simulink model "sistemas_mecanicos_simulink_simscape"  (R2025b)
settings: Solver=ode23t  StartTime=0.0  StopTime=10  RelTol=1e-3
libraries: fl_lib x21, nesl_utility x8
settings Model: Creator=Lenovo  LastModifiedBy=Lenovo

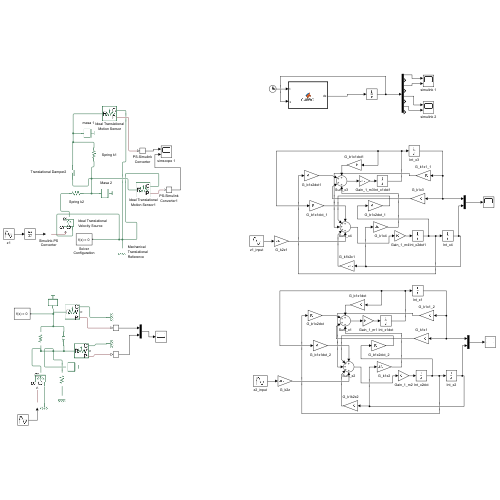
[thumbnail: Simulink's stored preview of the top-level diagram]
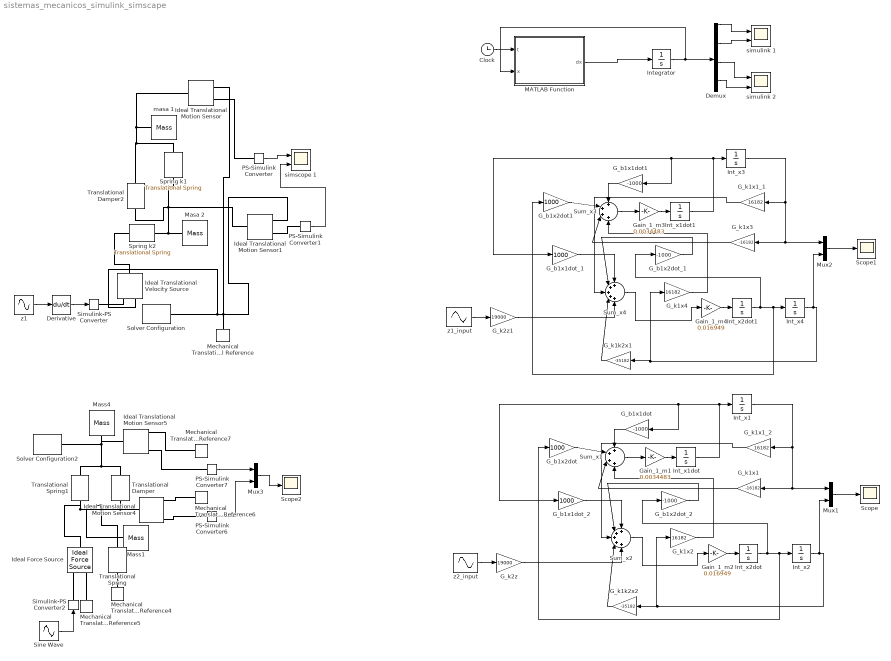
== system sistemas_mecanicos_simulink_simscape ==
  " Spring k1" : fl_lib/Mechanical/Translational Elements/Translational Spring  spr_rate=16182 N/m  v_specify=off  v_priority=None  v=0 m/s  v_nominal_specify=off  v_nominal_value=1  v_nominal_unit=m/s  f_specify=off  f_priority=None  f=0 N  f_nominal_specify=off  f_nominal_value=1  f_nominal_unit=N  x_specify=off  x_priority=High  x=0 m  x_nominal_specify=off  x_nominal_value=1  x_nominal_unit=m
  " Spring k2" : fl_lib/Mechanical/Translational Elements/Translational Spring  spr_rate=19000 N/m  v_specify=off  v_priority=None  v=0 m/s  v_nominal_specify=off  v_nominal_value=1  v_nominal_unit=m/s  f_specify=off  f_priority=None  f=0 N  f_nominal_specify=off  f_nominal_value=1  f_nominal_unit=N  x_specify=off  x_priority=High  x=0 m  x_nominal_specify=off  x_nominal_value=1  x_nominal_unit=m
  Clock : Clock
  Demux : Demux  Outputs=8
  Derivative : Derivative
  G_b1x1dot : Gain  Gain=-1000
  G_b1x1dot1 : Gain  Gain=-1000
  G_b1x1dot_1 : Gain  Gain=1000
  G_b1x1dot_2 : Gain  Gain=1000
  G_b1x2dot : Gain  Gain=1000
  G_b1x2dot1 : Gain  Gain=1000
  G_b1x2dot_1 : Gain  Gain=-1000
  G_b1x2dot_2 : Gain  Gain=-1000
  G_k1k2x1 : Gain  Gain=-35182
  G_k1k2x2 : Gain  Gain=-35182
  G_k1x1 : Gain  Gain=-16182
  G_k1x1_1 : Gain  Gain=16182
  G_k1x1_2 : Gain  Gain=16182
  G_k1x2 : Gain  Gain=16182
  G_k1x3 : Gain  Gain=-16182
  G_k1x4 : Gain  Gain=16182
  G_k2z : Gain  Gain=19000
  G_k2z1 : Gain  Gain=19000
  Gain_1_m1 : Gain  Gain=0.0034483
  Gain_1_m2 : Gain  Gain=0.016949
  Gain_1_m3 : Gain  Gain=0.0034483
  Gain_1_m4 : Gain  Gain=0.016949
  Ideal Force Source : fl_lib/Mechanical/Mechanical Sources/Ideal Force Source
  Ideal Translational Motion Sensor : fl_lib/Mechanical/Mechanical Sensors/Ideal Translational Motion Sensor  reference=foundation.enum.MeasurementReference.difference  acceleration_port=false  velocity_port=false  position_port=true  offset=0 m
      settings: InternalSimscapePortConfiguration="{\"Bottom\":[],\"Left\":[{\"id\":\"R\",\"label\":\"R\",\"type\":\"foundation.mechanical.translational.translational\"}],\"Right\":[{\"id\":\"C\",\"label\":\"C\",\"type\":\"foundation.mechanical.translational.translational\"},{\"id\":\"P\",\"label\":\"P\",\"type\":\"output\"}],\"Top\":[]}"
  Ideal Translational Motion Sensor1 : fl_lib/Mechanical/Mechanical Sensors/Ideal Translational Motion Sensor  reference=foundation.enum.MeasurementReference.difference  acceleration_port=false  velocity_port=false  position_port=true  offset=0 m
      settings: InternalSimscapePortConfiguration="{\"Bottom\":[],\"Left\":[{\"id\":\"R\",\"label\":\"R\",\"type\":\"foundation.mechanical.translational.translational\"}],\"Right\":[{\"id\":\"C\",\"label\":\"C\",\"type\":\"foundation.mechanical.translational.translational\"},{\"id\":\"P\",\"label\":\"P\",\"type\":\"output\"}],\"Top\":[]}"
  Ideal Translational Motion Sensor4 : fl_lib/Mechanical/Mechanical Sensors/Ideal Translational Motion Sensor  reference=foundation.enum.MeasurementReference.difference  acceleration_port=false  velocity_port=true  position_port=true  offset=0 m
  Ideal Translational Motion Sensor5 : fl_lib/Mechanical/Mechanical Sensors/Ideal Translational Motion Sensor  reference=foundation.enum.MeasurementReference.difference  acceleration_port=false  velocity_port=true  position_port=true  offset=0 m
  Ideal Translational Velocity Source : fl_lib/Mechanical/Mechanical Sources/Ideal Translational Velocity Source
  Int_x{1..4} (4 alike) : Integrator
  Int_x1dot : Integrator
  Int_x1dot1 : Integrator
  Int_x2dot : Integrator
  Int_x2dot1 : Integrator
  Integrator : Integrator  InitialCondition=zeros(8,1)
  MATLAB Function : MATLAB Function  TreatAsAtomicUnit=on
  Masa 2 : fl_lib/Mechanical/Translational Elements/Mass  mass=59 kg  num_ports=foundation.enum.numPorts2.one  v_specify=off  v_priority=High  v=0 m/s  v_nominal_specify=off  v_nominal_value=1  v_nominal_unit=m/s  f_specify=off  f_priority=None  f=0 N  f_nominal_specify=off  f_nominal_value=1  f_nominal_unit=N
  Mass1 : fl_lib/Mechanical/Translational Elements/Mass  mass=59 kg  num_ports=foundation.enum.numPorts2.one  v_specify=on  v_priority=High  v=0 m/s  v_nominal_specify=off  v_nominal_value=1  v_nominal_unit=m/s  f_specify=off  f_priority=None  f=0 N  f_nominal_specify=off  f_nominal_value=1  f_nominal_unit=N
  Mass4 : fl_lib/Mechanical/Translational Elements/Mass  mass=290 kg  num_ports=foundation.enum.numPorts2.one  v_specify=on  v_priority=High  v=0 m/s  v_nominal_specify=off  v_nominal_value=1  v_nominal_unit=m/s  f_specify=off  f_priority=None  f=0 N  f_nominal_specify=off  f_nominal_value=1  f_nominal_unit=N
  Mechanical Translational Reference{,4..7} (5 alike) : fl_lib/Mechanical/Translational Elements/Mechanical Translational Reference
  Mux1 : Mux  Inputs=2
  Mux2 : Mux  Inputs=2
  Mux3 : Mux  Inputs=2
  PS-Simulink Converter : nesl_utility/PS-Simulink Converter  PhysicalDomain=network_engine_domain  SubClassName=ps_output  LeftPortType=input  RightPortType=output  PseudoPeriodic=off  Frequencies=[]  VectorFormat=inherit  Unit=m  AffineConversion=off
  PS-Simulink Converter1 : nesl_utility/PS-Simulink Converter  PhysicalDomain=network_engine_domain  SubClassName=ps_output  LeftPortType=input  RightPortType=output  PseudoPeriodic=off  Frequencies=[]  VectorFormat=inherit  Unit=m  AffineConversion=off
  PS-Simulink Converter6 : nesl_utility/PS-Simulink Converter  PhysicalDomain=network_engine_domain  SubClassName=ps_output  LeftPortType=input  RightPortType=output  PseudoPeriodic=off  Frequencies=[]  VectorFormat=inherit  Unit=inherit  AffineConversion=off
  PS-Simulink Converter7 : nesl_utility/PS-Simulink Converter  PhysicalDomain=network_engine_domain  SubClassName=ps_output  LeftPortType=input  RightPortType=output  PseudoPeriodic=off  Frequencies=[]  VectorFormat=inherit  Unit=inherit  AffineConversion=off
  Scope : Scope
      settings: ActiveDisplayYMinimum=-0.0083300356795225766  ActiveDisplayYMaximum=0.014166622667732392  DataLoggingVariableName=ScopeData5
  Scope1 : Scope
      settings: ActiveDisplayYMinimum=-1  ActiveDisplayYMaximum=1  DataLoggingVariableName=ScopeData6
  Scope2 : Scope
      settings: ActiveDisplayYMinimum=-4.3042403537439215E-7  ActiveDisplayYMaximum=7.0921287947327007E-7  DataLoggingVariableName=ScopeData4
  Simulink-PS Converter : nesl_utility/Simulink-PS Converter  PhysicalDomain=network_engine_domain  SubClassName=ps_input  LeftPortType=input  RightPortType=output  PseudoPeriodic=off  Frequencies=[]  NoiseDistribution=none  NoiseParameters=[]  Unit=m/s  AffineConversion=off  FilteringAndDerivatives=provide  SimscapeFilterOrder=1  InputFilterTimeConstant=0.001  UdotUserProvided=0
  Simulink-PS Converter2 : nesl_utility/Simulink-PS Converter  PhysicalDomain=network_engine_domain  SubClassName=ps_input  LeftPortType=input  RightPortType=output  PseudoPeriodic=off  Frequencies=[]  NoiseDistribution=none  NoiseParameters=[]  Unit=1  AffineConversion=off  FilteringAndDerivatives=provide  SimscapeFilterOrder=1  InputFilterTimeConstant=0.001  UdotUserProvided=0
  Sine Wave : Sin  Amplitude=.05  Frequency=20*pi  SampleTime=0
  Solver Configuration : nesl_utility/Solver Configuration  PhysicalDomain=network_engine_domain  SubClassName=solver  LeftPortType=input  RightPortType=generic  Tones=[]  Harmonics=[]  SimulateNoise=off  Profile=off  UseLocalSampling=off  EnableSwitchedLinearOptims=on  FrequencyDomain=off  UseCCode=off  RelTol=0.001  AbsTol=0.001  MinStep=1e-09  ToWorkspace=off  RevertToSquareIcSolve=off  NumHomotopyIterations=100  PhasorMode=off  PhasorModeNumHarmonics=1  ConsistencySolver=NEWTON_XTOL_AFTER_FTOL  IndexReductionMethod=DerivativeReplacement  DoDC=off  ResidualTolerance=1e-09  ConsistencyTolSource=GLOBAL  ConsistencyAbsTol=0.001  ConsistencyRelTol=0.001  ConsistencyTolFactor=0.001  UseLocalSolver=off  LocalSolverChoice=NE_BACKWARD_EULER_ADVANCER  ResolveIndetEquations=on  FunctionEvalNumThread=1  LocalSolverSampleTime=0.001  DoFixedCost=off  MaxNonlinIter=3  MaxModeIter=2  ComputeImpulses=off  ImpulseIterations=2  LinearAlgebra=auto  LinearAlgebraNumThread=0  EquationFormulation=NE_TIME_EF  DelaysMemoryBudget=1024  AutomaticFiltering=on  FilteringTimeConstant=0.001  PartitionStorageMethod=AS_NEEDED  PartitionMemoryBudget=1024  PartitionMethod=ROBUST  MultibodyUseLocalSolver=off  MultibodyLocalSolverChoice=ODE1  MultibodyLocalSolverSampleTime=0.001
  Solver Configuration2 : nesl_utility/Solver Configuration  PhysicalDomain=network_engine_domain  SubClassName=solver  LeftPortType=input  RightPortType=generic  Tones=[]  Harmonics=[]  SimulateNoise=off  Profile=off  UseLocalSampling=off  EnableSwitchedLinearOptims=on  FrequencyDomain=off  UseCCode=off  RelTol=0.001  AbsTol=0.001  MinStep=1e-09  ToWorkspace=off  RevertToSquareIcSolve=off  NumHomotopyIterations=100  PhasorMode=off  PhasorModeNumHarmonics=1  ConsistencySolver=NEWTON_XTOL_AFTER_FTOL  IndexReductionMethod=DerivativeReplacement  DoDC=off  ResidualTolerance=1e-09  ConsistencyTolSource=GLOBAL  ConsistencyAbsTol=0.001  ConsistencyRelTol=0.001  ConsistencyTolFactor=0.001  UseLocalSolver=off  LocalSolverChoice=NE_BACKWARD_EULER_ADVANCER  ResolveIndetEquations=on  FunctionEvalNumThread=1  LocalSolverSampleTime=0.001  DoFixedCost=off  MaxNonlinIter=3  MaxModeIter=2  ComputeImpulses=off  ImpulseIterations=2  LinearAlgebra=auto  LinearAlgebraNumThread=0  EquationFormulation=NE_TIME_EF  DelaysMemoryBudget=1024  AutomaticFiltering=on  FilteringTimeConstant=0.001  PartitionStorageMethod=AS_NEEDED  PartitionMemoryBudget=1024  PartitionMethod=ROBUST  MultibodyUseLocalSolver=off  MultibodyLocalSolverChoice=ODE1  MultibodyLocalSolverSampleTime=0.001
  Sum_x1 : Sum  Inputs=++++
  Sum_x2 : Sum  Inputs=+++++
  Sum_x3 : Sum  Inputs=++++
  Sum_x4 : Sum  Inputs=+++++
  Translational Damper : fl_lib/Mechanical/Translational Elements/Translational Damper  D=1000 N*s/m  v_specify=off  v_priority=None  v=0 m/s  v_nominal_specify=off  v_nominal_value=1  v_nominal_unit=m/s  f_specify=off  f_priority=None  f=0 N  f_nominal_specify=off  f_nominal_value=1  f_nominal_unit=N
  Translational Damper2 : fl_lib/Mechanical/Translational Elements/Translational Damper  D=1000 N*s/m  v_specify=off  v_priority=None  v=0 m/s  v_nominal_specify=off  v_nominal_value=1  v_nominal_unit=m/s  f_specify=off  f_priority=None  f=0 N  f_nominal_specify=off  f_nominal_value=1  f_nominal_unit=N
  Translational Spring : fl_lib/Mechanical/Translational Elements/Translational Spring  spr_rate=19000 N/m  v_specify=off  v_priority=None  v=0 m/s  v_nominal_specify=off  v_nominal_value=1  v_nominal_unit=m/s  f_specify=off  f_priority=None  f=0 N  f_nominal_specify=off  f_nominal_value=1  f_nominal_unit=N  x_specify=on  x_priority=High  x=0 m  x_nominal_specify=off  x_nominal_value=1  x_nominal_unit=m
  Translational Spring1 : fl_lib/Mechanical/Translational Elements/Translational Spring  spr_rate=16182 N/m  v_specify=off  v_priority=None  v=0 m/s  v_nominal_specify=off  v_nominal_value=1  v_nominal_unit=m/s  f_specify=off  f_priority=None  f=0 N  f_nominal_specify=off  f_nominal_value=1  f_nominal_unit=N  x_specify=on  x_priority=High  x=0 m  x_nominal_specify=off  x_nominal_value=1  x_nominal_unit=m
  masa 1 : fl_lib/Mechanical/Translational Elements/Mass  mass=290 kg  num_ports=foundation.enum.numPorts2.one  v_specify=off  v_priority=High  v=0 m/s  v_nominal_specify=off  v_nominal_value=1  v_nominal_unit=m/s  f_specify=off  f_priority=None  f=0 N  f_nominal_specify=off  f_nominal_value=1  f_nominal_unit=N
  simscope 1 : Scope  NumInputPorts=2
      settings: ActiveDisplayYMinimum=-0.070119559663336467  ActiveDisplayYMaximum=0.080680383834571739  DataLoggingVariableName=ScopeData2
  simulink 1 : Scope  NumInputPorts=2
      settings: ActiveDisplayYMinimum=-0.070245818947862623  ActiveDisplayYMaximum=0.080562382084598858
  simulink 2 : Scope  NumInputPorts=2
      settings: ActiveDisplayYMinimum=-0.0083045632247379323  ActiveDisplayYMaximum=0.014180469478740158
  z1 : Sin  Amplitude=0.05  Frequency=0.5*pi  SampleTime=0
  z1_input : Sin  Amplitude=0.05  Frequency=1.5708  SampleTime=0
  z2_input : Sin  Amplitude=0.05  Frequency=62.8319  SampleTime=0
  wires:
  Integrator/1 -> Demux/1, MATLAB Function/2(x)
  MATLAB Function/1(dx) -> Integrator/1
  Demux/1 -> simulink 1/1
  Demux/3 -> simulink 1/2
  Demux/5 -> simulink 2/1
  Demux/7 -> simulink 2/2
  z1/1 -> Derivative/1
  Derivative/1 -> Simulink-PS Converter/1
  PS-Simulink Converter/1 -> simscope 1/1
  PS-Simulink Converter1/1 -> simscope 1/2
  Clock/1 -> MATLAB Function/1(t)
  G_k1x1/1 -> Sum_x1/3
  G_k2z1/1 -> Sum_x4/5
  Gain_1_m2/1 -> Int_x2dot/1
  Int_x1dot/1 -> G_b1x1dot/1, G_b1x1dot_2/1, Int_x1/1
  Int_x2dot1/1 -> Int_x4/1, G_b1x2dot1/1, G_b1x2dot_1/1
  G_k2z/1 -> Sum_x2/5
  G_b1x2dot_1/1 -> Sum_x4/2
  z2_input/1 -> G_k2z/1
  G_b1x2dot_2/1 -> Sum_x2/2
  Gain_1_m3/1 -> Int_x1dot1/1
  Int_x1dot1/1 -> G_b1x1dot1/1, G_b1x1dot_1/1, Int_x3/1
  Sum_x1/1 -> Gain_1_m1/1
  G_k1x3/1 -> Sum_x3/3
  G_b1x1dot_2/1 -> Sum_x2/1
  Sum_x3/1 -> Gain_1_m3/1
  G_b1x1dot/1 -> Sum_x1/1
  G_b1x1dot_1/1 -> Sum_x4/1
  G_k1x4/1 -> Sum_x3/4
  Int_x2dot/1 -> Int_x2/1, G_b1x2dot/1, G_b1x2dot_2/1
  Gain_1_m4/1 -> Int_x2dot1/1
  Sum_x4/1 -> Gain_1_m4/1
  Mux1/1 -> Scope/1
  Int_x3/1 -> G_k1x3/1, Mux2/1, G_k1x1_1/1
  Mux2/1 -> Scope1/1
  G_b1x2dot/1 -> Sum_x1/2
  Gain_1_m1/1 -> Int_x1dot/1
  G_k1x1_1/1 -> Sum_x4/3
  G_k1k2x2/1 -> Sum_x2/4
  G_b1x1dot1/1 -> Sum_x3/1
  Int_x4/1 -> G_k1k2x1/1, G_k1x4/1, Mux2/2
  G_b1x2dot1/1 -> Sum_x3/2
  Int_x1/1 -> G_k1x1/1, Mux1/1, G_k1x1_2/1
  Sum_x2/1 -> Gain_1_m2/1
  Int_x2/1 -> G_k1k2x2/1, G_k1x2/1, Mux1/2
  G_k1k2x1/1 -> Sum_x4/4
  G_k1x1_2/1 -> Sum_x2/3
  G_k1x2/1 -> Sum_x1/4
  z1_input/1 -> G_k2z1/1
  Sine Wave/1 -> Simulink-PS Converter2/1
  Mux3/1 -> Scope2/1
  PS-Simulink Converter7/1 -> Mux3/1
  PS-Simulink Converter6/1 -> Mux3/2
  connections:
  " Spring k2"/RConn1 -- Ideal Translational Motion Sensor1/LConn1 -- " Spring k1"/LConn1 -- Translational Damper2/LConn1 -- Masa 2/LConn1
  Simulink-PS Converter/RConn1 -- Ideal Translational Velocity Source/RConn1
  Ideal Translational Velocity Source/LConn1 -- " Spring k2"/LConn1
  PS-Simulink Converter/LConn1 -- Ideal Translational Motion Sensor/RConn2
  PS-Simulink Converter1/LConn1 -- Ideal Translational Motion Sensor1/RConn2
  " Spring k1"/RConn1 -- Ideal Translational Motion Sensor/LConn1 -- masa 1/LConn1 -- Translational Damper2/RConn1
  Mechanical Translational Reference/LConn1 -- Solver Configuration/RConn1 -- Ideal Translational Velocity Source/RConn2 -- Ideal Translational Motion Sensor/RConn1 -- Ideal Translational Motion Sensor1/RConn1
  Ideal Translational Motion Sensor5/LConn1 -- Translational Spring1/RConn1 -- Translational Damper/RConn1 -- Solver Configuration2/RConn1 -- Mass4/LConn1
  Ideal Translational Motion Sensor4/LConn1 -- Translational Spring/LConn1 -- Mass1/LConn1 -- Ideal Force Source/LConn1 -- Translational Spring1/LConn1 -- Translational Damper/LConn1
  Translational Spring/RConn1 -- Mechanical Translational Reference4/LConn1
  Mechanical Translational Reference5/LConn1 -- Ideal Force Source/RConn2
  Mechanical Translational Reference6/LConn1 -- Ideal Translational Motion Sensor4/RConn1
  PS-Simulink Converter6/LConn1 -- Ideal Translational Motion Sensor4/RConn3
  Simulink-PS Converter2/RConn1 -- Ideal Force Source/RConn1
  PS-Simulink Converter7/LConn1 -- Ideal Translational Motion Sensor5/RConn3
  Mechanical Translational Reference7/LConn1 -- Ideal Translational Motion Sensor5/RConn1

== matlab function sistemas_mecanicos_simulink_simscape/MATLAB Function ==
  data: t input; dx output; x input
function dx = CARRO(t,x)

m1 = 290;
b1 = 1000;
m2 = 59;
k1 = 16182;
k2 = 19000;
f= 0; 

z1 = 0.05 * sin(0.5 * pi * t);
z2 = 0.05 * sin(20 * pi * t);

dx = zeros(8,1);

dx(1) = x(2);

dx(2) = ((f/m1) - (b1/m1)*x(2) + (b1/m1)*x(4) - (k1/m1)*x(1) + (k1/m1)*x(3) );

dx(3) = x(4);

dx(4) = ( (b1/m2)*x(2) - (b1/m2)*x(4) + (k1/m2)*x(1) - ((k1+k2)/m2)*x(3) ) + (k2/m2)*z1;

dx(5) = x(6);

dx(6) = ((f/m1) - (b1/m1)*x(6) + (b1/m1)*x(8) - (k1/m1)*x(5) + (k1/m1)*x(7) );

dx(7) = x(8);

dx(8) = ( (b1/m2)*x(6) - (b1/m2)*x(8) + (k1/m2)*x(5) - ((k1+k2)/m2)*x(7) -(f/m2) + (k2/m2)*z2);

end
